simulink model "pendulum"  (R2023a)
settings: Solver=VariableStepAuto  StartTime=0.0  StopTime=100  MaxStep=0.05  RelTol=1e-3
undefined symbols (not defined in the file): I
libraries: simulink_extras x4
settings Model: Creator=tanov  LastModifiedBy=tanov

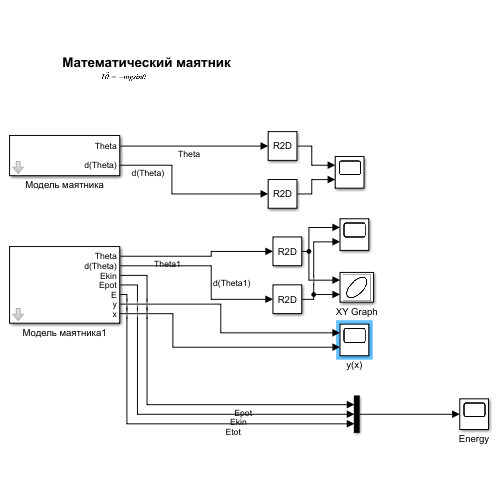
[thumbnail: Simulink's stored preview of the top-level diagram]
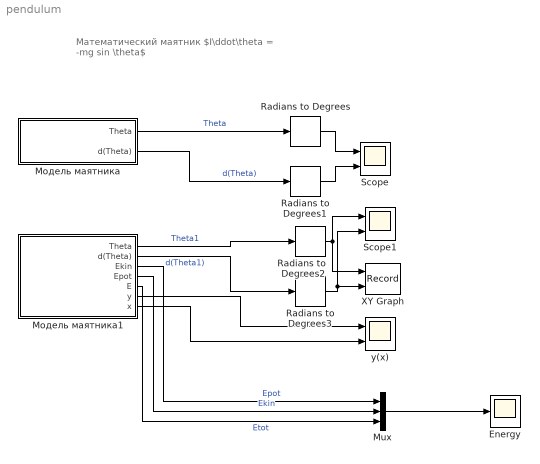
== system pendulum ==
  note: Математический маятник
      | $I\ddot\theta = -mg sin \theta$
  Energy : Scope
  Mux : Mux  Inputs=3
  Radians to Degrees{,1..3} (4 alike) : simulink_extras/Transformations/Radians to Degrees
  Scope : Scope  NumInputPorts=2
  Scope1 : Scope  NumInputPorts=2
  XY Graph : Record  FileSettingsInternal="{\"entries\":[{\"content\":{\"excelSettings\":{\"content\":{},\"type\":\"Streamout.ExcelSettings\"}},\"type\":\"Streamout.FileSettingStorage\",\"uuid\":\"ee290c55-a5fa-44ca-9fcd-6b3736a3a278\"}],\"packageUris\":[\"http://schema.mathworks.com/mf0/streamout_blocks/R2020a\"],\"version\":\"1.0\"}"  Layout=[1 1]  SignalsInternal="{\"entries\":[{\"content\":{\"signals\":[{\"content\":{\"blockPath\":[\"pendulum/XY Graph\"],\"dimensions\":[1],\"domain\":\"pendulum/XY Graph\",\"lineColor\":\"#a2142f\",\"plots\":[1],\"port\":1,\"sid\":[\"\"],\"signalID\":58,\"signalName\":\"Radians\\nto Degrees2\"},\"type\":\"RecordBlkView.Signal\",\"uuid\":\"a003e114-dbf8-4483-b388-096aa8d610e9\"},{\"content\":{\"blockPath\":[\"pendulum/XY Graph\"],\"dimensions\":[1],\"domain\":\"pendulum/XY Graph\",\"lineColor\":\"#139fff\",\"plots\":[1],\"port\":2,\"sid\":[\"\"],\"signalID\":62,\"signalName\":\"Radians\\nto Degrees3\"},\"type\":\"RecordBlkView.Signal\",\"uuid\":\"c59e1e9f-4330-4d48-a657-5aa3573eaadd\"}]},\"type\":\"RecordBlkView.InputSignals\",\"uuid\":\"7c4606bd-20bc-411f-985a-143776d547fe\"}],\"packageUris\":[\"http://schema.mathworks.com/mf0/streamout_blocks/R2020a\"],\"version\":\"1.0\"}"  VisualizationBindings="{\"xyplotplugin\":{\"info\":[{\"series\":[{\"bindingParametersList\":[{\"parameter\":\"X-Axis\",\"signalID\":58,\"signalName\":\"Radians\\nto Degrees2\"},{\"parameter\":\"Y-Axis\",\"signalID\":62,\"signalName\":\"Radians\\nto Degrees3\"}],\"seriesID\":3805}],\"subplotID\":1}]}}"  CompatibilityTag=XY
  y(x) : Scope  NumInputPorts=2
  Модель маятника : Subsystem  mask{m=2, L=1, g=9.8, startDegree=40}
      mask prompts: m "Масса"; L "Длина подвеса"; g "Угловая скорость"; startDegree "Начальный угол"
  Модель маятника1 : Subsystem  mask{m=1, L=1, g=9.8, startDegree=45, b=0.1}
      mask prompts: m "Масса"; L "Длина подвеса"; g "Угловая скорость"; startDegree "Начальный угол"; b "Коэффициент затухания"
  wires:
  Radians to Degrees/1 -> Scope/1
  Radians to Degrees1/1 -> Scope/2
  Модель маятника/1(Theta) -> Radians to Degrees/1  "Theta"
  Модель маятника/2(d(Theta)) -> Radians to Degrees1/1  "d(Theta)"
  Модель маятника1/2(d(Theta)) -> Radians to Degrees3/1  "d(Theta1)"
  Модель маятника1/1(Theta) -> Radians to Degrees2/1  "Theta1"
  Radians to Degrees3/1 -> XY Graph/2, Scope1/2
  Radians to Degrees2/1 -> XY Graph/1, Scope1/1
  Модель маятника1/6(y) -> y(x)/1
  Модель маятника1/7(x) -> y(x)/2
  Модель маятника1/3(Ekin) -> Mux/1  "Epot"
  Модель маятника1/4(Epot) -> Mux/2  "Ekin"
  Модель маятника1/5(E) -> Mux/3  "Etot"
  Mux/1 -> Energy/1

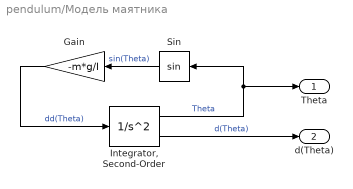
== system pendulum/Модель маятника ==
  Gain : Gain  Gain=-m*g/I
  "Integrator, Second-Order" : SecondOrderIntegrator  ICX=deg2rad(startDegree)
  Sin : Trigonometry
  Theta : Outport
  d(Theta) : Outport  Port=2
  wires:
  Sin/1 -> Gain/1  "sin(Theta)"
  Gain/1 -> "Integrator, Second-Order"/1  "dd(Theta)"
  "Integrator, Second-Order"/1 -> Theta/1, Sin/1  "Theta"
  "Integrator, Second-Order"/2 -> d(Theta)/1  "d(Theta)"

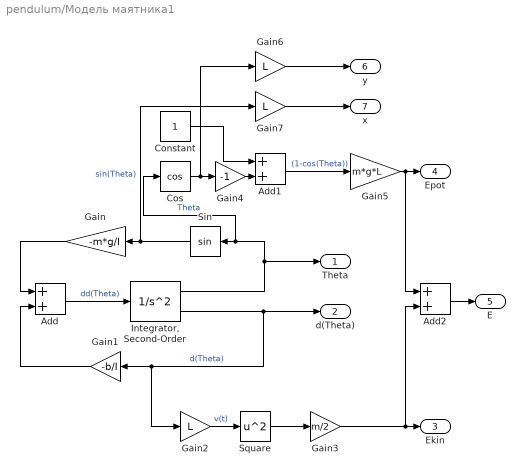
== system pendulum/Модель маятника1 ==
  Add : Sum
  Add1 : Sum
  Add2 : Sum
  Constant : Constant
  Cos : Trigonometry  Operator=cos
  Gain : Gain  Gain=-m*g/I
  Gain1 : Gain  Gain=-b/I
  Gain2 : Gain  Gain=L
  Gain3 : Gain  Gain=m/2
  Gain4 : Gain  Gain=-1
  Gain5 : Gain  Gain=m*g*L
  Gain6 : Gain  Gain=L
  Gain7 : Gain  Gain=L
  "Integrator, Second-Order" : SecondOrderIntegrator  ICX=deg2rad(startDegree)  ICDXDT=0
  Sin : Trigonometry
  Square : Math  Operator=square
  Theta : Outport
  d(Theta) : Outport  Port=2
  Ekin : Outport  Port=3
  Epot : Outport  Port=4
  E : Outport  Port=5
  y : Outport  Port=6
  x : Outport  Port=7
  wires:
  Sin/1 -> Gain/1, Gain7/1  "sin(Theta)"
  Gain/1 -> Add/1
  "Integrator, Second-Order"/1 -> Theta/1, Cos/1, Sin/1  "Theta"
  "Integrator, Second-Order"/2 -> Gain2/1, Gain1/1, d(Theta)/1  "d(Theta)"
  Add/1 -> "Integrator, Second-Order"/1  "dd(Theta)"
  Gain1/1 -> Add/2
  Gain2/1 -> Square/1  "v(t)"
  Square/1 -> Gain3/1
  Gain3/1 -> Add2/2, Ekin/1
  Cos/1 -> Gain6/1, Gain4/1
  Gain4/1 -> Add1/2
  Constant/1 -> Add1/1
  Add1/1 -> Gain5/1  "(1-cos(Theta))"
  Gain5/1 -> Add2/1, Epot/1
  Add2/1 -> E/1
  Gain6/1 -> y/1
  Gain7/1 -> x/1
